simulink model "siento_training_rt"  (Simulink 7.2)
settings: Solver=ode45  StartTime=0.0  StopTime=2  RelTol=1e-3
settings Model: Creator=rafa  LastModifiedBy=rafa

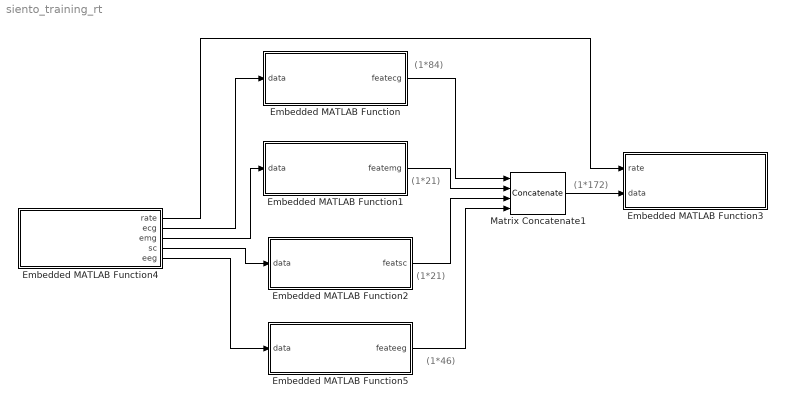
== system siento_training_rt ==
  note: (1*84)
  note: (1*21)
  note: (1*21)
  note: (1*172)
  note: (1*46)
  Embedded MATLAB Function : Stateflow chart
  Embedded MATLAB Function1 : Stateflow chart
  Embedded MATLAB Function2 : Stateflow chart
  Embedded MATLAB Function3 : Stateflow chart
  Embedded MATLAB Function4 : Stateflow chart
  Embedded MATLAB Function5 : Stateflow chart
  Matrix Concatenate1 : Concatenate  NumInputs=4  Mode=Multidimensional array
  wires:
  Embedded MATLAB Function/1(featecg) -> Matrix Concatenate1/1
  Embedded MATLAB Function1/1(featemg) -> Matrix Concatenate1/2
  Embedded MATLAB Function2/1(featsc) -> Matrix Concatenate1/3
  Matrix Concatenate1/1 -> Embedded MATLAB Function3/2(data)
  Embedded MATLAB Function4/2(ecg) -> Embedded MATLAB Function/1(data)
  Embedded MATLAB Function4/3(emg) -> Embedded MATLAB Function1/1(data)
  Embedded MATLAB Function4/4(sc) -> Embedded MATLAB Function2/1(data)
  Embedded MATLAB Function4/1(rate) -> Embedded MATLAB Function3/1(rate)
  Embedded MATLAB Function4/5(eeg) -> Embedded MATLAB Function5/1(data)
  Embedded MATLAB Function5/1(feateeg) -> Matrix Concatenate1/4

== matlab function Embedded MATLAB Function1 ==
  data: data input double; featemg output double
function featemg = emg_extract(data)
% This block supports the Embedded MATLAB subset.
% See the help menu for details. 
hz=1000;
if(min(data)==max(data))
    featvec=rand(1,21);
else
    featvec=zeros(1,21);
    featvec=feval('aubt_extractFeatEMG',data,hz);
end

featemg=featvec';

== matlab function Embedded MATLAB Function ==
  data: data input double; featecg output double
function featecg  = ecg_extract(data)
% This block supports the Embedded MATLAB subset.
% See the help menu for details. 
hz=1000;
if(min(data)==max(data))
    %when input constant, just sets feature vector to random numbers
    %to avoid errors
    featvec=rand(1,84);
    %featvec=feval('aubt_extractFeatECG',data,hz)
    %testing setup
    %featvec=[sum(data);rand(3,1)];
else
    featvec=rand(1,84);
    featvec=feval('aubt_extractFeatECG',data',hz);
end
featecg=featvec';

== matlab function Embedded MATLAB Function2 ==
  data: data input double; featsc output double
function featsc = sc_extract(data)
% This block supports the Embedded MATLAB subset.
% See the help menu for details. 
hz=1000;

if(min(data)==max(data))
    featvec=rand(1,21);
else
    featvec=zeros(1,21);
    featvec=feval('aubt_extractFeatSC',data,hz);
end

featsc=featvec';

== matlab function Embedded MATLAB Function3 ==
  data: rate input double; data input double
function   SaveAndFisherProject(rate,data)
% This block supports the Embedded MATLAB subset.
% See the help menu for details. 
data2=data';
rate2=rate';
feval('store',rate2,data2);
%feval('fisher_simulink',data2,rate2);

== matlab function Embedded MATLAB Function4 ==
  data: rate output double; ecg output double; emg output double; sc output double; eeg output double
function [rate,ecg,emg,sc,eeg]  = bioInput()
% This block supports the Embedded MATLAB subset.
% See the help menu for details. 
% if select==1 %simulation using mathematically generated signals
%         ecg=ecgGen(10);
%         emg=emgGen(10);
%         sc=scGen(10);
% end
% if select==2 %acquire signals from biopak
        ecg=zeros(1,10000);
        emg=zeros(1,10000);
        sc=zeros(1,10000);
        eeg=zeros(1,10000);
        rate=[0 0]';
        [rate,ecg,emg,sc,eeg]=feval('bioinput');
% end

== matlab function Embedded MATLAB Function5 ==
  data: data input double; feateeg output double
function feateeg = eeg_extract(data)
% This block supports the Embedded MATLAB subset.
% See the help menu for details. 
hz=1000;

if(min(data)==max(data))
    featvec=rand(1,58);
else
    featvec=zeros(1,58);
    featvec=feval('extractEEGFeatures2',data,hz);
end

feateeg=featvec';
